simulink subsystem "VehicleElectroThermal"  (R2024b)
settings: Solver=VariableStepAuto  StartTime=0.0  StopTime=10.0  RelTol=1e-3
undefined symbols (not defined in the file): coolant_pipe_D, coolant_valve_D_ratio_max, coolant_valve_D_ratio_min, coolant_valve_displacement, vehicleThermal
libraries: fl_lib x14, SimscapeFluids_lib x6, nesl_utility x6
(part 1 of 2)
Description:
  | This model represents an advanced Battery Electric Vehicle (BEV) architecture with integrated thermal management. It extends the basic electric drivetrain by modeling heat generation, transfer, and cooling subsystems for realistic thermal analysis.
  | 
  | Key Subsystems:
  | • Battery and dual electric motors (Front EM1 and Rear EM2)
  | • Driveline connecting front and rear axles for AWD operation
  | • Thermal components:
  |    - Heater and Chiller for thermal conditioning
  |    - Radiator for external heat rejection
  |    - Battery and Motor Pumps with coolant paths
  |    - Thermal valves and flow routing
  | • HVAC system and DCDC converter for cabin and auxiliary systems
  | • Charger interface for external power input
  | 
  | This Electro-Thermal model enables simulation of temperature effects on vehicle performance and energy consumption, making it ideal for thermal control development, range estimation under thermal load, and energy efficiency studies.
settings Model: Creator=jjha  LastModifiedBy=jjha
settings OptimizationCC: ReuseModelBlockBuffer=off
settings RTWCC: GPUComputeCapability=3.5

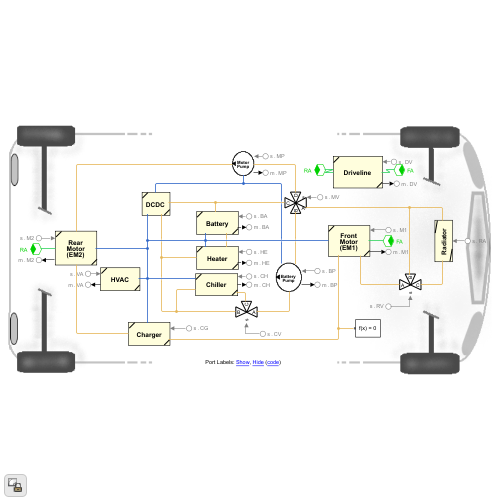
[thumbnail: Simulink's stored preview of the top-level diagram]
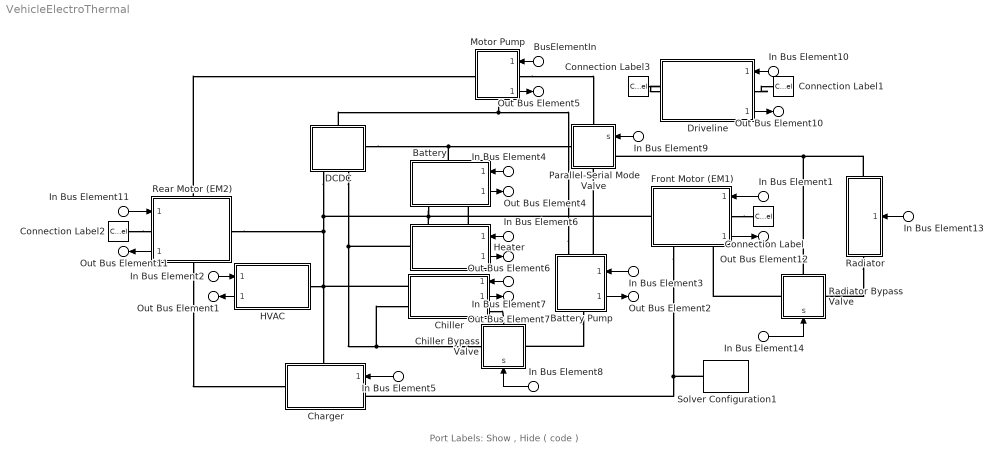
== system VehicleElectroThermal ==
  note: Port Labels: Show , Hide ( code )
  In Bus Element2 : Inport  PortName=s  Element=VA
  In Bus Element3 : Inport  PortName=s  Element=BP
  In Bus Element4 : Inport  PortName=s  Element=BA
  In Bus Element6 : Inport  PortName=s  Element=HE
  In Bus Element7 : Inport  PortName=s  Element=CH
  In Bus Element8 : Inport  PortName=s  Element=CV
  In Bus Element9 : Inport  PortName=s  Element=MV
  In Bus Element10 : Inport  PortName=s  Element=DV
  In Bus Element11 : Inport  PortName=s  Element=M2
  In Bus Element13 : Inport  PortName=s  Element=RA
  In Bus Element14 : Inport  PortName=s  Element=RV
  BusElementIn : Inport  PortName=s  Element=MP
  In Bus Element5 : Inport  PortName=s  Element=CG
  In Bus Element1 : Inport  PortName=s  Element=M1
  Battery : Subsystem  ReferencedSubsystem=BatteryTableBased
      settings: PortSchema="{\"entries\":[{\"content\":{\"sides\":[{\"content\":{\"connectorIds\":[\"In1\",\"Out1\"]},\"type\":\"ConnectorPlacement.EquallySpacedRectSide\",\"uuid\":\"8937d0fc-2bf4-4b6f-a857-82b384a76c94\"},{\"content\":{\"side\":\"RIGHT\"},\"type\":\"ConnectorPlacement.EquallySpacedRectSide\",\"uuid\":\"1ccbeec6-a013-4076-9f98-cb308866a19c\"},{\"content\":{\"connectorIds\":[\"LConn1\"],\"side\":\"TOP\"},\"type\":\"ConnectorPlacement.EquallySpacedRectSide\",\"uuid\":\"77a454e3-c37c-480e-9dd0-9550186f5eb3\"},{\"content\":{\"connectorIds\":[\"RConn1\",\"RConn2\"],\"side\":\"BOTTOM\"},\"type\":\"ConnectorPlacement.EquallySpacedRectSide\",\"uuid\":\"f9a87c6a-7374-41c2-a5df-89d60c915a70\"}]},\"type\":\"ConnectorPlacement.EquallySpacedConnector\",\"uuid\":\"fe008494-fd6d-45a8-bf6b-36872afbad95\"}],\"packageUris\":[\"http://schema.mathworks.com/mf0/Connector/R2020b\"],\"version\":\"1.0\"}"
  Battery Pump : Subsystem  ReferencedSubsystem=Pump  pump_displacement=pump.pump_displacement  pump_speed_max=pump.pump_speed_max  coolant_pipe_D=pump.coolant_pipe_D
      settings: PortSchema="{\"entries\":[{\"content\":{\"sides\":[{\"content\":{\"connectorIds\":[\"In1\",\"Out1\"]},\"type\":\"ConnectorPlacement.EquallySpacedRectSide\",\"uuid\":\"f321ff85-78a4-45a4-ab97-f20c5abfaf5e\"},{\"content\":{\"side\":\"RIGHT\"},\"type\":\"ConnectorPlacement.EquallySpacedRectSide\",\"uuid\":\"2baf3540-3ef2-4140-8c68-0a1895e3ee25\"},{\"content\":{\"connectorIds\":[\"LConn1\",\"LConn2\"],\"side\":\"TOP\"},\"type\":\"ConnectorPlacement.EquallySpacedRectSide\",\"uuid\":\"1e5b09ba-71c5-41d6-b265-2fb2d783e941\"},{\"content\":{\"connectorIds\":[\"RConn1\"],\"side\":\"BOTTOM\"},\"type\":\"ConnectorPlacement.EquallySpacedRectSide\",\"uuid\":\"e2f6a4b1-a05e-4597-9342-cdf640c5f71b\"}]},\"type\":\"ConnectorPlacement.EquallySpacedConnector\",\"uuid\":\"4c01441a-ee4a-4858-900a-4caacc6910c3\"}],\"packageUris\":[\"http://schema.mathworks.com/mf0/Connector/R2020b\"],\"version\":\"1.0\"}"
  Charger : Subsystem  ReferencedSubsystem=ChargerThermalDummy
      settings: PortSchema="{\"entries\":[{\"content\":{\"sides\":[{\"content\":{\"connectorIds\":[\"In1\",\"LConn1\"]},\"type\":\"ConnectorPlacement.EquallySpacedRectSide\",\"uuid\":\"cb45011f-5d5d-4b7e-92e7-7d115d1e4fd6\"},{\"content\":{\"connectorIds\":[\"RConn1\"],\"side\":\"RIGHT\"},\"type\":\"ConnectorPlacement.EquallySpacedRectSide\",\"uuid\":\"cd67087d-6bbf-411e-9f50-cc3c1f5fce85\"},{\"content\":{\"connectorIds\":[\"LConn2\"],\"side\":\"TOP\"},\"type\":\"ConnectorPlacement.EquallySpacedRectSide\",\"uuid\":\"32ff64c9-862a-431f-9f24-2baf455cdab5\"}]},\"type\":\"ConnectorPlacement.EquallySpacedConnector\",\"uuid\":\"13ffd7d0-36a1-4766-a9dc-2d010b2a8713\"}],\"packageUris\":[\"http://schema.mathworks.com/mf0/Connector/R2020b\"],\"version\":\"1.0\"}"
  Chiller : Subsystem  ReferencedSubsystem=Chiller
      settings: PortSchema="{\"entries\":[{\"content\":{\"sides\":[{\"content\":{\"connectorIds\":[\"LConn1\",\"LConn2\"]},\"type\":\"ConnectorPlacement.EquallySpacedRectSide\",\"uuid\":\"5c01cf01-1aa7-4ead-a658-6b31c847d37c\"},{\"content\":{\"connectorIds\":[\"In1\",\"Out1\",\"RConn1\"],\"side\":\"RIGHT\"},\"type\":\"ConnectorPlacement.EquallySpacedRectSide\",\"uuid\":\"fa598d46-0793-4efa-a9e2-c958f5dfdee6\"},{\"content\":{\"side\":\"TOP\"},\"type\":\"ConnectorPlacement.EquallySpacedRectSide\",\"uuid\":\"e82d971a-2580-41ee-87fa-0ab5603b5665\"},{\"content\":{\"side\":\"BOTTOM\"},\"type\":\"ConnectorPlacement.EquallySpacedRectSide\",\"uuid\":\"431a910f-738f-40ab-a4d4-f974d0793b92\"}]},\"type\":\"ConnectorPlacement.EquallySpacedConnector\",\"uuid\":\"9f63eeb1-1768-47e0-a5e5-2e43c100d3fd\"}],\"packageUris\":[\"http://schema.mathworks.com/mf0/Connector/R2020b\"],\"version\":\"1.0\"}"
  Chiller Bypass Valve : Subsystem  Tag=PublishSubsystem
      settings: PortSchema="{\"entries\":[{\"content\":{\"sides\":[{\"content\":{\"connectorIds\":[\"LConn1\"]},\"type\":\"ConnectorPlacement.EquallySpacedRectSide\",\"uuid\":\"3cf8f321-e6af-4e16-922c-cceb23b0b295\"},{\"content\":{\"connectorIds\":[\"In1\"],\"side\":\"RIGHT\"},\"type\":\"ConnectorPlacement.EquallySpacedRectSide\",\"uuid\":\"d134eacd-e7eb-4b63-940a-90eaf4978625\"},{\"content\":{\"connectorIds\":[\"LConn2\"],\"side\":\"TOP\"},\"type\":\"ConnectorPlacement.EquallySpacedRectSide\",\"uuid\":\"57a3d5f7-3b46-4166-b258-196ae00f6810\"},{\"content\":{\"connectorIds\":[\"RConn1\"],\"side\":\"BOTTOM\"},\"type\":\"ConnectorPlacement.EquallySpacedRectSide\",\"uuid\":\"637149da-33c2-49a6-af44-c757a7002402\"}]},\"type\":\"ConnectorPlacement.EquallySpacedConnector\",\"uuid\":\"8ee22012-655b-4352-9f09-996f74687633\"}],\"packageUris\":[\"http://schema.mathworks.com/mf0/Connector/R2020b\"],\"version\":\"1.0\"}"
      mask Display:
      | color('white')
      | plot(100, 100)
      | plot(-100, -100)
      | color('black')
      | 
      | plot([0 -100 -100 0], [0 50 -50 0])
      | plot([0 50 -50 0], [0 100 100 0])
      | plot([0 50 -50 0], [0 -100 -100 0])
  Connection Label : ConnectionLabel  Label=FA
  Connection Label1 : ConnectionLabel  Label=FA
  Connection Label2 : ConnectionLabel  Label=RA
  Connection Label3 : ConnectionLabel  Label=RA
  DCDC : Subsystem  ReferencedSubsystem=PumpDriverTh
      settings: PortSchema="{\"entries\":[{\"content\":{\"sides\":[{\"content\":{\"connectorIds\":[\"RConn2\"]},\"type\":\"ConnectorPlacement.EquallySpacedRectSide\",\"uuid\":\"8937d0fc-2bf4-4b6f-a857-82b384a76c94\"},{\"content\":{\"side\":\"RIGHT\"},\"type\":\"ConnectorPlacement.EquallySpacedRectSide\",\"uuid\":\"1ccbeec6-a013-4076-9f98-cb308866a19c\"},{\"content\":{\"connectorIds\":[\"RConn1\"],\"side\":\"TOP\"},\"type\":\"ConnectorPlacement.EquallySpacedRectSide\",\"uuid\":\"77a454e3-c37c-480e-9dd0-9550186f5eb3\"},{\"content\":{\"connectorIds\":[\"LConn2\",\"LConn1\"],\"side\":\"BOTTOM\"},\"type\":\"ConnectorPlacement.EquallySpacedRectSide\",\"uuid\":\"f9a87c6a-7374-41c2-a5df-89d60c915a70\"}]},\"type\":\"ConnectorPlacement.EquallySpacedConnector\",\"uuid\":\"fe008494-fd6d-45a8-bf6b-36872afbad95\"}],\"packageUris\":[\"http://schema.mathworks.com/mf0/Connector/R2020b\"],\"version\":\"1.0\"}"
  Driveline : Subsystem  ReferencedSubsystem=Driveline
      settings: PortSchema="{\"entries\":[{\"content\":{\"sides\":[{\"content\":{\"connectorIds\":[\"In1\",\"LConn1\",\"Out1\"]},\"type\":\"ConnectorPlacement.EquallySpacedRectSide\",\"uuid\":\"f321ff85-78a4-45a4-ab97-f20c5abfaf5e\"},{\"content\":{\"connectorIds\":[\"RConn1\"],\"side\":\"RIGHT\"},\"type\":\"ConnectorPlacement.EquallySpacedRectSide\",\"uuid\":\"2baf3540-3ef2-4140-8c68-0a1895e3ee25\"},{\"content\":{\"side\":\"TOP\"},\"type\":\"ConnectorPlacement.EquallySpacedRectSide\",\"uuid\":\"1e5b09ba-71c5-41d6-b265-2fb2d783e941\"}]},\"type\":\"ConnectorPlacement.EquallySpacedConnector\",\"uuid\":\"4c01441a-ee4a-4858-900a-4caacc6910c3\"}],\"packageUris\":[\"http://schema.mathworks.com/mf0/Connector/R2020b\"],\"version\":\"1.0\"}"
  Front Motor (EM1) : Subsystem  ReferencedSubsystem=MotorDriveGearTh  max_torque=electricDrive.max_torque  max_power=electricDrive.max_power  Tctc=electricDrive.Tctc  motor_loss_map=electricDrive.motor_loss_map  coolant_channel_D=electricDrive.coolant_channel_D
      settings: PortSchema="{\"entries\":[{\"content\":{\"sides\":[{\"content\":{\"connectorIds\":[\"In1\",\"RConn1\",\"Out1\"]},\"type\":\"ConnectorPlacement.EquallySpacedRectSide\",\"uuid\":\"af07bd2d-3590-42bb-89c7-c9779cf31117\"},{\"content\":{\"connectorIds\":[\"LConn1\"],\"side\":\"RIGHT\"},\"type\":\"ConnectorPlacement.EquallySpacedRectSide\",\"uuid\":\"06bccd0a-b2e1-4e74-ae56-c1e69a7ba035\"},{\"content\":{\"side\":\"TOP\"},\"type\":\"ConnectorPlacement.EquallySpacedRectSide\",\"uuid\":\"3cab1049-b411-40ea-b5ea-dc5d5d9a0e66\"},{\"content\":{\"connectorIds\":[\"LConn2\",\"RConn2\"],\"side\":\"BOTTOM\"},\"type\":\"ConnectorPlacement.EquallySpacedRectSide\",\"uuid\":\"a1b63549-7d05-436f-845e-36a4f25eae53\"}]},\"type\":\"ConnectorPlacement.EquallySpacedConnector\",\"uuid\":\"d2f6dabd-9c76-4b80-9c91-dda4599c36e7\"}],\"packageUris\":[\"http://schema.mathworks.com/mf0/Connector/R2020b\"],\"version\":\"1.0\"}"
  HVAC : Subsystem  ReferencedSubsystem=HVACsimpleTh
      settings: PortSchema="{\"entries\":[{\"content\":{\"sides\":[{\"content\":{\"connectorIds\":[\"LConn1\"]},\"type\":\"ConnectorPlacement.EquallySpacedRectSide\",\"uuid\":\"f3199610-b7b9-4772-9d43-f46decbe6ee9\"},{\"content\":{\"connectorIds\":[\"In1\",\"Out1\"],\"side\":\"RIGHT\"},\"type\":\"ConnectorPlacement.EquallySpacedRectSide\",\"uuid\":\"92399d3a-435b-4545-8fb9-2408b0c62154\"},{\"content\":{\"side\":\"TOP\"},\"type\":\"ConnectorPlacement.EquallySpacedRectSide\",\"uuid\":\"9d5257be-bcde-46da-a005-cbe35149e50d\"},{\"content\":{\"side\":\"BOTTOM\"},\"type\":\"ConnectorPlacement.EquallySpacedRectSide\",\"uuid\":\"da7f19de-1e57-4fc2-b5c3-4c1d680ac086\"}]},\"type\":\"ConnectorPlacement.EquallySpacedConnector\",\"uuid\":\"aa27bbb1-a774-4836-83ea-faf9e12779cd\"}],\"packageUris\":[\"http://schema.mathworks.com/mf0/Connector/R2020b\"],\"version\":\"1.0\"}"
  Heater : Subsystem  ReferencedSubsystem=Heater
      settings: PortSchema="{\"entries\":[{\"content\":{\"sides\":[{\"content\":{},\"type\":\"ConnectorPlacement.EquallySpacedRectSide\",\"uuid\":\"f321ff85-78a4-45a4-ab97-f20c5abfaf5e\"},{\"content\":{\"connectorIds\":[\"RConn1\",\"RConn2\"],\"side\":\"RIGHT\"},\"type\":\"ConnectorPlacement.EquallySpacedRectSide\",\"uuid\":\"2baf3540-3ef2-4140-8c68-0a1895e3ee25\"},{\"content\":{\"connectorIds\":[\"Out1\",\"In1\"],\"side\":\"TOP\"},\"type\":\"ConnectorPlacement.EquallySpacedRectSide\",\"uuid\":\"1e5b09ba-71c5-41d6-b265-2fb2d783e941\"},{\"content\":{\"connectorIds\":[\"RConn3\"],\"side\":\"BOTTOM\"},\"type\":\"ConnectorPlacement.EquallySpacedRectSide\",\"uuid\":\"2993c442-350f-4391-ac34-e98798b669d5\"}]},\"type\":\"ConnectorPlacement.EquallySpacedConnector\",\"uuid\":\"4c01441a-ee4a-4858-900a-4caacc6910c3\"}],\"packageUris\":[\"http://schema.mathworks.com/mf0/Connector/R2020b\"],\"version\":\"1.0\"}"
  Motor Pump : Subsystem  ReferencedSubsystem=Pump  pump_displacement=pump.pump_displacement  pump_speed_max=pump.pump_speed_max  coolant_pipe_D=pump.coolant_pipe_D
      settings: PortSchema="{\"entries\":[{\"content\":{\"sides\":[{\"content\":{\"connectorIds\":[\"In1\",\"LConn1\",\"Out1\"]},\"type\":\"ConnectorPlacement.EquallySpacedRectSide\",\"uuid\":\"f321ff85-78a4-45a4-ab97-f20c5abfaf5e\"},{\"content\":{\"connectorIds\":[\"RConn1\"],\"side\":\"RIGHT\"},\"type\":\"ConnectorPlacement.EquallySpacedRectSide\",\"uuid\":\"2baf3540-3ef2-4140-8c68-0a1895e3ee25\"},{\"content\":{\"side\":\"TOP\"},\"type\":\"ConnectorPlacement.EquallySpacedRectSide\",\"uuid\":\"1e5b09ba-71c5-41d6-b265-2fb2d783e941\"},{\"content\":{\"connectorIds\":[\"LConn2\"],\"side\":\"BOTTOM\"},\"type\":\"ConnectorPlacement.EquallySpacedRectSide\",\"uuid\":\"e2f6a4b1-a05e-4597-9342-cdf640c5f71b\"}]},\"type\":\"ConnectorPlacement.EquallySpacedConnector\",\"uuid\":\"4c01441a-ee4a-4858-900a-4caacc6910c3\"}],\"packageUris\":[\"http://schema.mathworks.com/mf0/Connector/R2020b\"],\"version\":\"1.0\"}"
  Parallel-Serial Mode Valve : Subsystem  Tag=PublishSubsystem
      settings: PortSchema="{\"entries\":[{\"content\":{\"sides\":[{\"content\":{\"connectorIds\":[\"LConn1\"]},\"type\":\"ConnectorPlacement.EquallySpacedRectSide\",\"uuid\":\"37aeff26-8a07-411b-9eeb-30a57d0de01e\"},{\"content\":{\"connectorIds\":[\"RConn1\"],\"side\":\"RIGHT\"},\"type\":\"ConnectorPlacement.EquallySpacedRectSide\",\"uuid\":\"5bec464c-49bf-4ce7-bef9-f1dcc380cec5\"},{\"content\":{\"connectorIds\":[\"LConn2\",\"In1\"],\"side\":\"TOP\"},\"type\":\"ConnectorPlacement.EquallySpacedRectSide\",\"uuid\":\"af2a9b5d-b1fd-40d4-a7a1-24f37b8a323f\"},{\"content\":{\"connectorIds\":[\"RConn2\"],\"side\":\"BOTTOM\"},\"type\":\"ConnectorPlacement.EquallySpacedRectSide\",\"uuid\":\"7361a3ef-1473-4ec0-bd8f-80e79015a6c8\"}]},\"type\":\"ConnectorPlacement.EquallySpacedConnector\",\"uuid\":\"019cf393-57f8-4763-b38e-2892ad46a0e9\"}],\"packageUris\":[\"http://schema.mathworks.com/mf0/Connector/R2020b\"],\"version\":\"1.0\"}"
      mask Display:
      | color('white')
      | plot(100, 100)
      | plot(-100, -100)
      | color('black')
      | 
      | plot([0 -100 -100 0], [0 50 -50 0])
      | plot([0 100 100 0], [0 50 -50 0])
      | plot([0 50 -50 0], [0 100 100 0])
      | plot([0 50 -50 0], [0 -100 -100 0])
  Radiator : Subsystem  ReferencedSubsystem=Radiator
      settings: PortSchema="{\"entries\":[{\"content\":{\"sides\":[{\"content\":{\"connectorIds\":[\"RConn1\"]},\"type\":\"ConnectorPlacement.EquallySpacedRectSide\",\"uuid\":\"af07bd2d-3590-42bb-89c7-c9779cf31117\"},{\"content\":{\"connectorIds\":[\"LConn1\"],\"side\":\"RIGHT\"},\"type\":\"ConnectorPlacement.EquallySpacedRectSide\",\"uuid\":\"06bccd0a-b2e1-4e74-ae56-c1e69a7ba035\"},{\"content\":{\"connectorIds\":[\"In1\"],\"side\":\"TOP\"},\"type\":\"ConnectorPlacement.EquallySpacedRectSide\",\"uuid\":\"3cab1049-b411-40ea-b5ea-dc5d5d9a0e66\"},{\"content\":{\"side\":\"BOTTOM\"},\"type\":\"ConnectorPlacement.EquallySpacedRectSide\",\"uuid\":\"a1b63549-7d05-436f-845e-36a4f25eae53\"}]},\"type\":\"ConnectorPlacement.EquallySpacedConnector\",\"uuid\":\"d2f6dabd-9c76-4b80-9c91-dda4599c36e7\"}],\"packageUris\":[\"http://schema.mathworks.com/mf0/Connector/R2020b\"],\"version\":\"1.0\"}"
  Radiator Bypass Valve : Subsystem  Tag=PublishSubsystem
      settings: PortSchema="{\"entries\":[{\"content\":{\"sides\":[{\"content\":{\"connectorIds\":[\"LConn1\"]},\"type\":\"ConnectorPlacement.EquallySpacedRectSide\",\"uuid\":\"3cf8f321-e6af-4e16-922c-cceb23b0b295\"},{\"content\":{\"connectorIds\":[\"In1\"],\"side\":\"RIGHT\"},\"type\":\"ConnectorPlacement.EquallySpacedRectSide\",\"uuid\":\"d134eacd-e7eb-4b63-940a-90eaf4978625\"},{\"content\":{\"connectorIds\":[\"LConn2\"],\"side\":\"TOP\"},\"type\":\"ConnectorPlacement.EquallySpacedRectSide\",\"uuid\":\"57a3d5f7-3b46-4166-b258-196ae00f6810\"},{\"content\":{\"connectorIds\":[\"RConn1\"],\"side\":\"BOTTOM\"},\"type\":\"ConnectorPlacement.EquallySpacedRectSide\",\"uuid\":\"f8aa24a3-5169-478a-b161-4d226dc0f508\"}]},\"type\":\"ConnectorPlacement.EquallySpacedConnector\",\"uuid\":\"8ee22012-655b-4352-9f09-996f74687633\"}],\"packageUris\":[\"http://schema.mathworks.com/mf0/Connector/R2020b\"],\"version\":\"1.0\"}"
      mask Display:
      | color('white')
      | plot(100, 100)
      | plot(-100, -100)
      | color('black')
      | 
      | plot([0 -100 -100 0], [0 50 -50 0])
      | plot([0 50 -50 0], [0 100 100 0])
      | plot([0 50 -50 0], [0 -100 -100 0])
  Rear Motor (EM2) : Subsystem  ReferencedSubsystem=MotorDriveGearTh  max_torque=electricDrive.max_torque  max_power=electricDrive.max_power  Tctc=electricDrive.Tctc  motor_loss_map=electricDrive.motor_loss_map  coolant_channel_D=electricDrive.coolant_channel_D
      settings: PortSchema="{\"entries\":[{\"content\":{\"sides\":[{\"content\":{\"connectorIds\":[\"In1\",\"RConn1\",\"Out1\"]},\"type\":\"ConnectorPlacement.EquallySpacedRectSide\",\"uuid\":\"af07bd2d-3590-42bb-89c7-c9779cf31117\"},{\"content\":{\"connectorIds\":[\"LConn1\"],\"side\":\"RIGHT\"},\"type\":\"ConnectorPlacement.EquallySpacedRectSide\",\"uuid\":\"06bccd0a-b2e1-4e74-ae56-c1e69a7ba035\"},{\"content\":{\"connectorIds\":[\"LConn2\"],\"side\":\"TOP\"},\"type\":\"ConnectorPlacement.EquallySpacedRectSide\",\"uuid\":\"3cab1049-b411-40ea-b5ea-dc5d5d9a0e66\"},{\"content\":{\"connectorIds\":[\"RConn2\"],\"side\":\"BOTTOM\"},\"type\":\"ConnectorPlacement.EquallySpacedRectSide\",\"uuid\":\"a1b63549-7d05-436f-845e-36a4f25eae53\"}]},\"type\":\"ConnectorPlacement.EquallySpacedConnector\",\"uuid\":\"d2f6dabd-9c76-4b80-9c91-dda4599c36e7\"}],\"packageUris\":[\"http://schema.mathworks.com/mf0/Connector/R2020b\"],\"version\":\"1.0\"}"
  Solver Configuration1 : nesl_utility/Solver Configuration  PhysicalDomain=network_engine_domain  SubClassName=solver  LeftPortType=input  RightPortType=generic  Tones=[]  Harmonics=[]  SimulateNoise=off  Profile=off  UseLocalSampling=off  EnableSwitchedLinearOptims=on  FrequencyDomain=off  UseCCode=off  RelTol=0.001  AbsTol=0.001  MinStep=1e-09  ToWorkspace=off  RevertToSquareIcSolve=off  NumHomotopyIterations=100  PhasorMode=off  PhasorModeNumHarmonics=1  ConsistencySolver=NEWTON_XTOL_AFTER_FTOL  IndexReductionMethod=DerivativeReplacement  DoDC=off  ResidualTolerance=1e-09  ConsistencyTolSource=GLOBAL  ConsistencyAbsTol=0.001  ConsistencyRelTol=0.001  ConsistencyTolFactor=0.001  UseLocalSolver=off  LocalSolverChoice=NE_BACKWARD_EULER_ADVANCER  ResolveIndetEquations=on  FunctionEvalNumThread=1  LocalSolverSampleTime=0.001  DoFixedCost=off  MaxNonlinIter=3  MaxModeIter=2  ComputeImpulses=off  ImpulseIterations=2  LinearAlgebra=auto  LinearAlgebraNumThread=0  EquationFormulation=NE_TIME_EF  DelaysMemoryBudget=1024  AutomaticFiltering=on  FilteringTimeConstant=0.001  PartitionStorageMethod=AS_NEEDED  PartitionMemoryBudget=1024  PartitionMethod=ROBUST  MultibodyUseLocalSolver=off  MultibodyLocalSolverChoice=ODE1  MultibodyLocalSolverSampleTime=0.001
  Out Bus Element1 : Outport  PortName=m  Element=VA
  Out Bus Element2 : Outport  PortName=m  Element=BP
  Out Bus Element4 : Outport  PortName=m  Element=BA
  Out Bus Element6 : Outport  PortName=m  Element=HE
  Out Bus Element7 : Outport  PortName=m  Element=CH
  Out Bus Element10 : Outport  PortName=m  Element=DV
  Out Bus Element11 : Outport  PortName=m  Element=M2
  Out Bus Element12 : Outport  PortName=m  Element=M1
  Out Bus Element5 : Outport  PortName=m  Element=MP
  wires:
  In Bus Element2/1 -> HVAC/1
  In Bus Element6/1 -> Heater/1
  In Bus Element4/1 -> Battery/1
  Chiller/1 -> Out Bus Element7/1
  In Bus Element7/1 -> Chiller/1
  Battery Pump/1 -> Out Bus Element2/1
  BusElementIn/1 -> Motor Pump/1
  In Bus Element3/1 -> Battery Pump/1
  Battery/1 -> Out Bus Element4/1
  HVAC/1 -> Out Bus Element1/1
  In Bus Element8/1 -> Chiller Bypass Valve/1(s)
  In Bus Element9/1 -> Parallel-Serial Mode Valve/1(s)
  Driveline/1 -> Out Bus Element10/1
  In Bus Element10/1 -> Driveline/1
  In Bus Element11/1 -> Rear Motor (EM2)/1
  Rear Motor (EM2)/1 -> Out Bus Element11/1
  Front Motor (EM1)/1 -> Out Bus Element12/1
  In Bus Element13/1 -> Radiator/1
  In Bus Element14/1 -> Radiator Bypass Valve/1(s)
  In Bus Element5/1 -> Charger/1
  Heater/1 -> Out Bus Element6/1
  Motor Pump/1 -> Out Bus Element5/1
  In Bus Element1/1 -> Front Motor (EM1)/1
  connections:
  Radiator Bypass Valve/LConn1 -- Parallel-Serial Mode Valve/LConn2 -- Radiator/LConn1
  Front Motor (EM1)/RConn2 -- Charger/LConn1 -- Solver Configuration1/RConn1
  Chiller Bypass Valve/RConn1 -- DCDC/LConn2 -- Heater/RConn3 -- Chiller/LConn2
  DCDC/RConn2 -- Parallel-Serial Mode Valve/RConn2 -- Battery/LConn1
  Front Motor (EM1)/LConn1 -- Chiller/LConn1 -- Charger/LConn2 -- HVAC/LConn1 -- Rear Motor (EM2)/LConn1 -- DCDC/LConn1 -- Heater/RConn2 -- Battery/RConn2
  Battery Pump/LConn2 -- DCDC/RConn1 -- Motor Pump/LConn2
  Battery Pump/RConn1 -- Chiller Bypass Valve/LConn2
  Motor Pump/LConn1 -- Parallel-Serial Mode Valve/RConn1
  Rear Motor (EM2)/LConn2 -- Motor Pump/RConn1
  Battery Pump/LConn1 -- Parallel-Serial Mode Valve/LConn1
  Rear Motor (EM2)/RConn2 -- Charger/RConn1
  Front Motor (EM1)/RConn1 -- Connection Label/LConn1
  Chiller/RConn1 -- Chiller Bypass Valve/LConn1
  Radiator/RConn1 -- Radiator Bypass Valve/RConn1
  Driveline/LConn1 -- Connection Label1/LConn1
  Connection Label3/LConn1 -- Driveline/RConn1
  Heater/RConn1 -- Battery/RConn1
  Radiator Bypass Valve/LConn2 -- Front Motor (EM1)/LConn2
  Connection Label2/LConn1 -- Rear Motor (EM2)/RConn1

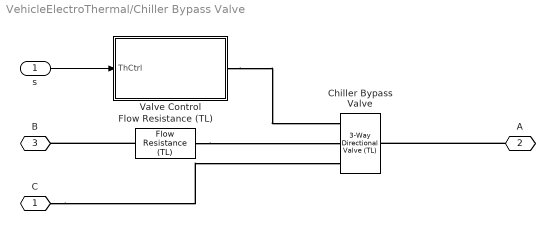
== system VehicleElectroThermal/Chiller Bypass Valve ==
  s : Inport
  Chiller Bypass Valve : SimscapeFluids_lib/Thermal Liquid/Valves & Orifices/Directional Control Valves/3-Way Directional Valve (TL)  open_orifices_pos=fluids.thermal_liquid.valves.directional_control_valves.enum.OpenOrifices3Way.PA  open_orifices_neg=fluids.thermal_liquid.valves.directional_control_valves.enum.OpenOrifices3Way.AT  area_spec=fluids.thermal_liquid.valves.directional_control_valves.enum.area_spec.identical  valve_spec=fluids.thermal_liquid.valves.enum.orifice_spec.linear  del_S_max=vehicleThermal.coolant_valve_displacement-(vehicleThermal.coolant_valve_displacement)*(pi * (vehicleThermal.coolant_valve_D_ratio_min*vehicleThermal.coolant_pipe_D)^2 / 4)/(pi * (vehicleThermal.coolant_valve_D_ratio_max*vehicleThermal.coolant_pipe_D)^2 / 4) m  area_max=pi * (vehicleThermal.coolant_valve_D_ratio_max*vehicleThermal.coolant_pipe_D)^2 / 4 m^2  del_S_TLU=[0 0.002 0.004 0.007 0.017] m  valve_area_TLU=[1e-09, 2.0352e-07, 4.0736e-05, .00011438, .00034356] m^2  del_S_flow_TLU=[0 0.002 0.004 0.007 0.017] m  p_diff_TLU=[-.1, .3, .5, .7] MPa  vol_flow_TLU=1e-3 * [1.7e-05, 2e-05, 2.6e-05; .0035, .0045, .0053; .7, .9, 1.06; 1.96, 2.5, 3; 6, 7.7, 9.13] m^3/s  mdot_TLU=[-1e-05, 1.7e-05, 2e-05, 2.6e-05; -.002, .0035, .0045, .0053; -.4, .7, .9, 1.06; -1.13, 1.96, 2.5, 3; -3.45, 6, 7.7, 9.13] kg/s  T_ref_in=293.15 K  p_ref_in=0.101325 MPa  area_leak=pi * (vehicleThermal.coolant_valve_D_ratio_min*vehicleThermal.coolant_pipe_D)^2 / 4 m^2  Cd=0.7  Re_c=12  smoothing_factor=0.01  pressure_recovery=simscape.enum.onoff.on  area=pi * vehicleThermal.coolant_pipe_D^2 / 4 m^2  S_max_PA=(vehicleThermal.coolant_valve_displacement)*(pi * (vehicleThermal.coolant_valve_D_ratio_min*vehicleThermal.coolant_pipe_D)^2 / 4)/(pi * (vehicleThermal.coolant_valve_D_ratio_max*vehicleThermal.coolant_pipe_D)^2 / 4) - (vehicleThermal.coolant_valve_offset) + vehicleThermal.coolant_valve_displacement-(vehicleThermal.coolant_valve_displacement)*(pi * (vehicleThermal.coolant_valve_D_ratio_min*vehicleThermal.coolant_pipe_D)^2 / 4)/(pi * (vehicleThermal.coolant_valve_D_ratio_max*vehicleThermal.coolant_pipe_D)^2 / 4) m  del_S_max_PA=coolant_valve_displacement-(coolant_valve_displacement)*(pi * (coolant_valve_D_ratio_min*coolant_pipe_D)^2 / 4)/(pi * (coolant_valve_D_ratio_max*coolant_pipe_D)^2 / 4) m  area_max_PA=pi * (coolant_valve_D_ratio_max*coolant_pipe_D)^2 / 4 m^2  del_S_TLU_PA=[0 0.002 0.004 0.007 0.017] m  valve_area_TLU_PA=[1e-09, 2.0352e-07, 4.0736e-05, .00011438, .00034356] m^2  del_S_flow_TLU_PA=[0 0.002 0.004 0.007 0.017] m  p_diff_TLU_PA=[-.1, .3, .5, .7] MPa  vol_flow_TLU_PA=1e-3 * [1.7e-05, 2e-05, 2.6e-05; .0035, .0045, .0053; .7, .9, 1.06; 1.96, 2.5, 3; 6, 7.7, 9.13] m^3/s  mdot_TLU_PA=[-1e-05, 1.7e-05, 2e-05, 2.6e-05; -.002, .0035, .0045, .0053; -.4, .7, .9, 1.06; -1.13, 1.96, 2.5, 3; -3.45, 6, 7.7, 9.13] kg/s  S_max_AT=-(vehicleThermal.coolant_valve_displacement)*(pi * (vehicleThermal.coolant_valve_D_ratio_min*vehicleThermal.coolant_pipe_D)^2 / 4)/(pi * (vehicleThermal.coolant_valve_D_ratio_max*vehicleThermal.coolant_pipe_D)^2 / 4) + (vehicleThermal.coolant_valve_offset) - (vehicleThermal.coolant_valve_displacement-(vehicleThermal.coolant_valve_displacement)*(pi * (vehicleThermal.coolant_valve_D_ratio_min*vehicleThermal.coolant_pipe_D)^2 / 4)/(pi * (vehicleThermal.coolant_valve_D_ratio_max*vehicleThermal.coolant_pipe_D)^2 / 4)) m  del_S_max_AT=coolant_valve_displacement-(coolant_valve_displacement)*(pi * (coolant_valve_D_ratio_min*coolant_pipe_D)^2 / 4)/(pi * (coolant_valve_D_ratio_max*coolant_pipe_D)^2 / 4) m  area_max_AT=pi * (coolant_valve_D_ratio_max*coolant_pipe_D)^2 / 4 m^2  del_S_TLU_AT=[0 0.002 0.004 0.007 0.017] m  valve_area_TLU_AT=[1e-09, 2.0352e-07, 4.0736e-05, .00011438, .00034356] m^2  del_S_flow_TLU_AT=[0 0.002 0.004 0.007 0.017] m  p_diff_TLU_AT=[-.1, .3, .5, .7] MPa  vol_flow_TLU_AT=1e-3 * [1.7e-05, 2e-05, 2.6e-05; .0035, .0045, .0053; .7, .9, 1.06; 1.96, 2.5, 3; 6, 7.7, 9.13] m^3/s  mdot_TLU_AT=[-1e-05, 1.7e-05, 2e-05, 2.6e-05; -.002, .0035, .0045, .0053; -.4, .7, .9, 1.06; -1.13, 1.96, 2.5, 3; -3.45, 6, 7.7, 9.13] kg/s  S_max_PT=2.5e-3 m  del_S_max_PT=0.005 m  area_max_PT=1e-4 m^2  del_S_TLU_PT=[0, .002, .004, .007, .017] m  valve_area_TLU_PT=[1e-09, 2.0352e-07, 4.0736e-05, .00011438, .00034356] m^2  del_S_flow_TLU_PT=[0, .002, .004, .007, .017] m  p_diff_TLU_PT=[.3, .5, .7] MPa  vol_flow_TLU_PT=1e-3 * [1.7e-05, 2e-05, 2.6e-05; .0035, .0045, .0053; .7, .9, 1.06; 1.96, 2.5, 3; 6, 7.7, 9.13] m^3/s  mdot_TLU_PT=[1.7e-05, 2e-05, 2.6e-05; .0035, .0045, .0053; .7, .9, 1.06; 1.96, 2.5, 3; 6, 7.7, 9.13] kg/s
      settings: InternalSimscapePortConfiguration="{\"Bottom\":[],\"Left\":[{\"id\":\"A\",\"label\":\"A\",\"type\":\"foundation.thermal_liquid.thermal_liquid\"}],\"Right\":[{\"id\":\"S\",\"label\":\"S\",\"type\":\"input\"},{\"id\":\"P\",\"label\":\"P\",\"type\":\"foundation.thermal_liquid.thermal_liquid\"},{\"id\":\"T\",\"label\":\"T\",\"type\":\"foundation.thermal_liquid.thermal_liquid\"}],\"Top\":[]}"
  Flow Resistance (TL) : fl_lib/Thermal Liquid/Elements/Flow Resistance (TL)  delta_p_nominal=0.001 MPa  mdot_nominal=0.3 kg/s  area=pi * vehicleThermal.coolant_pipe_D^2 / 4 m^2  laminar_fraction=1e-3
  Valve Control : Subsystem
  C : PMIOPort  Side=Left
  A : PMIOPort  Port=2  Side=Left
  B : PMIOPort  Port=3  Side=Right
  wires:
  s/1 -> Valve Control/1(ThCtrl)
  connections:
  Flow Resistance (TL)/LConn1 -- Chiller Bypass Valve/RConn2
  A/RConn1 -- Chiller Bypass Valve/LConn1
  Valve Control/RConn1 -- Chiller Bypass Valve/RConn1
  C/RConn1 -- Chiller Bypass Valve/RConn3
  Flow Resistance (TL)/RConn1 -- B/RConn1

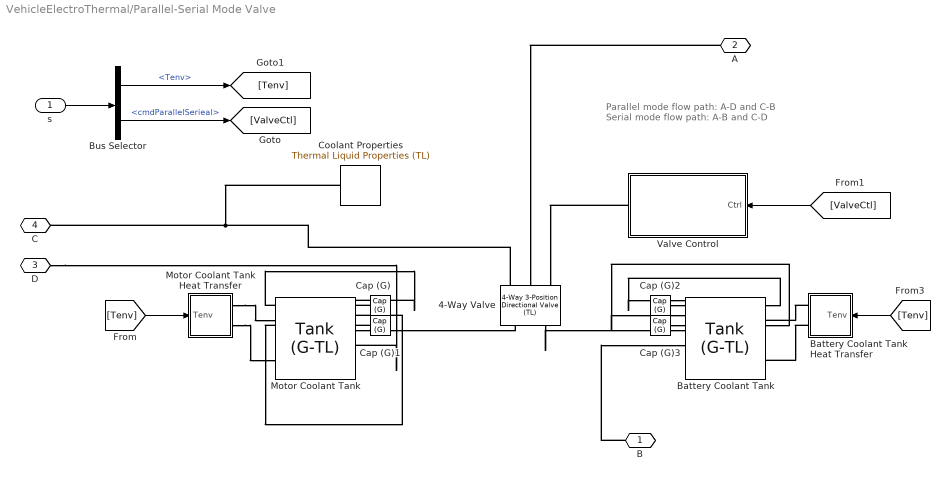
== system VehicleElectroThermal/Parallel-Serial Mode Valve ==
  note: Parallel mode flow path: A-D and C-B
      |
      | Serial mode flow path: A-B and C-D
  s : Inport
  4-Way Valve : SimscapeFluids_lib/Thermal Liquid/Valves & Orifices/Directional Control Valves/4-Way 3-Position Directional Valve (TL)  open_orifices_pos=fluids.thermal_liquid.valves.directional_control_valves.enum.OpenOrifices4WayPosNeg.PA_BT  open_orifices_neu=fluids.thermal_liquid.valves.directional_control_valves.enum.OpenOrifices4WayNeu.all_closed  open_orifices_neg=fluids.thermal_liquid.valves.directional_control_valves.enum.OpenOrifices4WayPosNeg.PB_AT  neutral_assert_action=simscape.enum.assert.action.none  area_spec=fluids.thermal_liquid.valves.directional_control_valves.enum.area_spec.identical  valve_spec=fluids.thermal_liquid.valves.enum.orifice_spec.linear  del_S_max=vehicleThermal.coolant_valve_displacement-(vehicleThermal.coolant_valve_displacement)*(pi * (vehicleThermal.coolant_valve_D_ratio_min*vehicleThermal.coolant_pipe_D)^2 / 4)/(pi * (vehicleThermal.coolant_valve_D_ratio_max*vehicleThermal.coolant_pipe_D)^2 / 4) m  area_max=pi * (vehicleThermal.coolant_valve_D_ratio_max*vehicleThermal.coolant_pipe_D)^2 / 4 m^2  del_S_TLU=[0 0.002 0.004 0.007 0.017] m  valve_area_TLU=[1e-09, 2.0352e-07, 4.0736e-05, .00011438, .00034356] m^2  del_S_flow_TLU=[0 0.002 0.004 0.007 0.017] m  p_diff_TLU=[-.1, .3, .5, .7] MPa  vol_flow_TLU=[-1e-08, 2.2e-08, 2.8e-08, 3.4e-08; -9e-06, .00015, .0002, .00024; -.00036, .00063, .00081, .00096; -.00054, .00094, .0012, .0014; -.00091, .0016, .002, .0024] m^3/s  mdot_TLU=[-1e-05, 1.7e-05, 2e-05, 2.6e-05; -.002, .0035, .0045, .0053; -.4, .7, .9, 1.06; -1.13, 1.96, 2.5, 3; -3.45, 6, 7.7, 9.13] kg/s  p_diff_TLU_const=[-.1, .3, .5, .7] MPa  vol_flow_TLU_const=[-.0009, .0016, .002, .0024] m^3/s  mdot_TLU_const=[-.9, 1.6, 2, 2.4] kg/s  area_const=1e-4 m^2  T_ref_in=293.15 K  p_ref_in=0.101325 MPa  area_leak=pi * (vehicleThermal.coolant_valve_D_ratio_min*vehicleThermal.coolant_pipe_D)^2 / 4 m^2  area=pi * vehicleThermal.coolant_pipe_D^2 / 4 m^2  Cd=0.7  Re_c=12  smoothing_factor=0.01  pressure_recovery=simscape.enum.onoff.on  S_max_PA=(vehicleThermal.coolant_valve_displacement)*(pi * (vehicleThermal.coolant_valve_D_ratio_min*vehicleThermal.coolant_pipe_D)^2 / 4)/(pi * (vehicleThermal.coolant_valve_D_ratio_max*vehicleThermal.coolant_pipe_D)^2 / 4) - (vehicleThermal.coolant_valve_offset) + vehicleThermal.coolant_valve_displacement-(vehicleThermal.coolant_valve_displacement)*(pi * (vehicleThermal.coolant_valve_D_ratio_min*vehicleThermal.coolant_pipe_D)^2 / 4)/(pi * (vehicleThermal.coolant_valve_D_ratio_max*vehicleThermal.coolant_pipe_D)^2 / 4) m  del_S_max_PA=coolant_valve_displacement-(coolant_valve_displacement)*(pi * (coolant_valve_D_ratio_min*coolant_pipe_D)^2 / 4)/(pi * (coolant_valve_D_ratio_max*coolant_pipe_D)^2 / 4) m  area_max_PA=pi * (coolant_valve_D_ratio_max*coolant_pipe_D)^2 / 4 m^2  del_S_TLU_PA=[0 0.002 0.004 0.007 0.017] m  valve_area_TLU_PA=[1e-09, 2.0352e-07, 4.0736e-05, .00011438, .00034356] m^2  del_S_flow_TLU_PA=[0 0.002 0.004 0.007 0.017] m  p_diff_TLU_PA=[-.1, .3, .5, .7] MPa  vol_flow_TLU_PA=[-1e-08, 2.2e-08, 2.8e-08, 3.4e-08; -9e-06, .00015, .0002, .00024; -.00036, .00063, .00081, .00096; -.00054, .00094, .0012, .0014; -.00091, .0016, .002, .0024] m^3/s  mdot_TLU_PA=[-1e-05, 1.7e-05, 2e-05, 2.6e-05; -.002, .0035, .0045, .0053; -.4, .7, .9, 1.06; -1.13, 1.96, 2.5, 3; -3.45, 6, 7.7, 9.13] kg/s  area_const_PA=1e-4 m^2  p_diff_TLU_const_PA=[-.1, .3, .5, .7] MPa  vol_flow_TLU_const_PA=[-.0009, .0016, .002, .0024] m^3/s  mdot_TLU_const_PA=[-.9, 1.6, 2, 2.4] kg/s  S_max_PB=-(vehicleThermal.coolant_valve_displacement)*(pi * (vehicleThermal.coolant_valve_D_ratio_min*vehicleThermal.coolant_pipe_D)^2 / 4)/(pi * (vehicleThermal.coolant_valve_D_ratio_max*vehicleThermal.coolant_pipe_D)^2 / 4) + (vehicleThermal.coolant_valve_offset) - (vehicleThermal.coolant_valve_displacement-(vehicleThermal.coolant_valve_displacement)*(pi * (vehicleThermal.coolant_valve_D_ratio_min*vehicleThermal.coolant_pipe_D)^2 / 4)/(pi * (vehicleThermal.coolant_valve_D_ratio_max*vehicleThermal.coolant_pipe_D)^2 / 4)) m  del_S_max_PB=coolant_valve_displacement-(coolant_valve_displacement)*(pi * (coolant_valve_D_ratio_min*coolant_pipe_D)^2 / 4)/(pi * (coolant_valve_D_ratio_max*coolant_pipe_D)^2 / 4) m  area_max_PB=pi * (coolant_valve_D_ratio_max*coolant_pipe_D)^2 / 4 m^2  del_S_TLU_PB=[0 0.002 0.004 0.007 0.017] m  valve_area_TLU_PB=[1e-09, 2.0352e-07, 4.0736e-05, .00011438, .00034356] m^2  del_S_flow_TLU_PB=[0 0.002 0.004 0.007 0.017] m  p_diff_TLU_PB=[-.1, .3, .5, .7] MPa  vol_flow_TLU_PB=[-1e-08, 2.2e-08, 2.8e-08, 3.4e-08; -9e-06, .00015, .0002, .00024; -.00036, .00063, .00081, .00096; -.00054, .00094, .0012, .0014; -.00091, .0016, .002, .0024] m^3/s  mdot_TLU_PB=[-1e-05, 1.7e-05, 2e-05, 2.6e-05; -.002, .0035, .0045, .0053; -.4, .7, .9, 1.06; -1.13, 1.96, 2.5, 3; -3.45, 6, 7.7, 9.13] kg/s  area_const_PB=1e-4 m^2  p_diff_TLU_const_PB=[-.1, .3, .5, .7] MPa  vol_flow_TLU_const_PB=[-.0009, .0016, .002, .0024] m^3/s  mdot_TLU_const_PB=[-.9, 1.6, 2, 2.4] kg/s  S_max_AB=7.5e-3 m  del_S_max_AB=0.005 m  area_max_AB=1e-4 m^2  del_S_TLU_AB=[0, .00125, .0025, .00375, .005] m  valve_area_TLU_AB=[1e-10, 1e-05, 4e-05, 6e-05, .0001] m^2  del_S_flow_TLU_AB=[0, .00125, .0025, .00375, .005] m  p_diff_TLU_AB=[-.1, .3, .5, .7] MPa  vol_flow_TLU_AB=[-1e-08, 2.2e-08, 2.8e-08, 3.4e-08; -9e-06, .00015, .0002, .00024; -.00036, .00063, .00081, .00096; -.00054, .00094, .0012, .0014; -.00091, .0016, .002, .0024] m^3/s  mdot_TLU_AB=[-1e-05, 1.7e-05, 2e-05, 2.6e-05; -.009, .0035, .0045, .0053; -.36, .7, .9, 1.06; -.54, 1.96, 2.5, 3; -.91, 6, 7.7, 9.13] kg/s  area_const_AB=1e-4 m^2  p_diff_TLU_const_AB=[-.1, .3, .5, .7] MPa  vol_flow_TLU_const_AB=[-.0009, .0016, .002, .0024] m^3/s  mdot_TLU_const_AB=[-.9, 1.6, 2, 2.4] kg/s  S_max_AT=-(vehicleThermal.coolant_valve_displacement)*(pi * (vehicleThermal.coolant_valve_D_ratio_min*vehicleThermal.coolant_pipe_D)^2 / 4)/(pi * (vehicleThermal.coolant_valve_D_ratio_max*vehicleThermal.coolant_pipe_D)^2 / 4) + (vehicleThermal.coolant_valve_offset) - (vehicleThermal.coolant_valve_displacement-(vehicleThermal.coolant_valve_displacement)*(pi * (vehicleThermal.coolant_valve_D_ratio_min*vehicleThermal.coolant_pipe_D)^2 / 4)/(pi * (vehicleThermal.coolant_valve_D_ratio_max*vehicleThermal.coolant_pipe_D)^2 / 4)) m  del_S_max_AT=coolant_valve_displacement-(coolant_valve_displacement)*(pi * (coolant_valve_D_ratio_min*coolant_pipe_D)^2 / 4)/(pi * (coolant_valve_D_ratio_max*coolant_pipe_D)^2 / 4) m  area_max_AT=pi * (coolant_valve_D_ratio_max*coolant_pipe_D)^2 / 4 m^2  del_S_TLU_AT=[0 0.002 0.004 0.007 0.017] m  valve_area_TLU_AT=[1e-09, 2.0352e-07, 4.0736e-05, .00011438, .00034356] m^2  del_S_flow_TLU_AT=[0 0.002 0.004 0.007 0.017] m  p_diff_TLU_AT=[-.1, .3, .5, .7] MPa  vol_flow_TLU_AT=[-1e-08, 2.2e-08, 2.8e-08, 3.4e-08; -9e-06, .00015, .0002, .00024; -.00036, .00063, .00081, .00096; -.00054, .00094, .0012, .0014; -.00091, .0016, .002, .0024] m^3/s  mdot_TLU_AT=[-1e-05, 1.7e-05, 2e-05, 2.6e-05; -.002, .0035, .0045, .0053; -.4, .7, .9, 1.06; -1.13, 1.96, 2.5, 3; -3.45, 6, 7.7, 9.13] kg/s  area_const_AT=1e-4 m^2  p_diff_TLU_const_AT=[-.1, .3, .5, .7] MPa  vol_flow_TLU_const_AT=[-.0009, .0016, .002, .0024] m^3/s  mdot_TLU_const_AT=[-.9, 1.6, 2, 2.4] kg/s  S_max_BT=(vehicleThermal.coolant_valve_displacement)*(pi * (vehicleThermal.coolant_valve_D_ratio_min*vehicleThermal.coolant_pipe_D)^2 / 4)/(pi * (vehicleThermal.coolant_valve_D_ratio_max*vehicleThermal.coolant_pipe_D)^2 / 4) - (vehicleThermal.coolant_valve_offset) + vehicleThermal.coolant_valve_displacement-(vehicleThermal.coolant_valve_displacement)*(pi * (vehicleThermal.coolant_valve_D_ratio_min*vehicleThermal.coolant_pipe_D)^2 / 4)/(pi * (vehicleThermal.coolant_valve_D_ratio_max*vehicleThermal.coolant_pipe_D)^2 / 4) m  del_S_max_BT=coolant_valve_displacement-(coolant_valve_displacement)*(pi * (coolant_valve_D_ratio_min*coolant_pipe_D)^2 / 4)/(pi * (coolant_valve_D_ratio_max*coolant_pipe_D)^2 / 4) m  area_max_BT=pi * (coolant_valve_D_ratio_max*coolant_pipe_D)^2 / 4 m^2  del_S_TLU_BT=[0 0.002 0.004 0.007 0.017] m  valve_area_TLU_BT=[1e-09, 2.0352e-07, 4.0736e-05, .00011438, .00034356] m^2  del_S_flow_TLU_BT=[0 0.002 0.004 0.007 0.017] m  p_diff_TLU_BT=[-.1, .3, .5, .7] MPa  vol_flow_TLU_BT=[-1e-08, 2.2e-08, 2.8e-08, 3.4e-08; -9e-06, .00015, .0002, .00024; -.00036, .00063, .00081, .00096; -.00054, .00094, .0012, .0014; -.00091, .0016, .002, .0024] m^3/s  mdot_TLU_BT=[-1e-05, 1.7e-05, 2e-05, 2.6e-05; -.002, .0035, .0045, .0053; -.4, .7, .9, 1.06; -1.13, 1.96, 2.5, 3; -3.45, 6, 7.7, 9.13] kg/s  area_const_BT=1e-4 m^2  p_diff_TLU_const_BT=[-.1, .3, .5, .7] MPa  vol_flow_TLU_const_BT=[-.0009, .0016, .002, .0024] m^3/s  mdot_TLU_const_BT=[-.9, 1.6, 2, 2.4] kg/s  S_max_PT=0 m  del_S_max_PT=0.005 m  area_max_PT=1e-4 m^2  del_S_TLU_PT=[0, .00125, .0025, .00375, .005] m  valve_area_TLU_PT=[1e-10, 1e-05, 4e-05, 6e-05, .0001] m^2  del_S_flow_TLU_PT=[0, .00125, .0025, .00375, .005] m  p_diff_TLU_PT=[-.1, .3, .5, .7] MPa  vol_flow_TLU_PT=[-1e-08, 2.2e-08, 2.8e-08, 3.4e-08; -9e-06, .00015, .0002, .00024; -.00036, .00063, .00081, .00096; -.00054, .00094, .0012, .0014; -.00091, .0016, .002, .0024] m^3/s  mdot_TLU_PT=[-1e-05, 1.7e-05, 2e-05, 2.6e-05; -.009, .0035, .0045, .0053; -.36, .7, .9, 1.06; -.54, 1.96, 2.5, 3; -.91, 6, 7.7, 9.13] kg/s
      settings: InternalSimscapePortConfiguration="{\"Bottom\":[],\"Left\":[{\"id\":\"A\",\"label\":\"A\",\"type\":\"foundation.thermal_liquid.thermal_liquid\"},{\"id\":\"B\",\"label\":\"B\",\"type\":\"foundation.thermal_liquid.thermal_liquid\"}],\"Right\":[{\"id\":\"S\",\"label\":\"S\",\"type\":\"input\"},{\"id\":\"P\",\"label\":\"P\",\"type\":\"foundation.thermal_liquid.thermal_liquid\"},{\"id\":\"T\",\"label\":\"T\",\"type\":\"foundation.thermal_liquid.thermal_liquid\"}],\"Top\":[]}"
  Battery Coolant Tank : SimscapeFluids_lib/Thermal Liquid/Tanks & Accumulators/Tank (G-TL)  num_inlet=2  volume_total=vehicleThermal.coolant_tank_volume l  volume_spec=1  tank_area=vehicleThermal.coolant_tank_area m^2  level_TLU=[0, 3, 5] m  volume_TLU=[0, 4, 6] m^3  inlet_areas_A1B1=[.01, .01] m^2  inlet_height_A2=0.1 m  inlet_area_A2=0.01 m^2  inlet_heights_A2B2=[0, 0] m  inlet_areas_A2B2=[1 1] * pi * vehicleThermal.coolant_pipe_D^2 / 4 m^2  inlet_heights_A2B2C2=[.1, .1, .1] m  inlet_areas_A2B2C2=[.01, .01, .01] m^2  inlet_heights_A2B2C2D2=0.1 * ones(1, 4) m  inlet_areas_A2B2C2D2=0.01 * ones(1, 4) m^2  inlet_heights_A2B2C2D2E2=0.1 * ones(1, 5) m  inlet_areas_A2B2C2D2E2=0.01 * ones(1, 5) m^2  inlet_heights_A2B2C2D2E2F2=0.1 * ones(1, 6) m  inlet_areas_A2B2C2D2E2F2=0.01 * ones(1, 6) m^2  capacity_check=0  max_liquid_capacity=vehicleThermal.coolant_tank_volume l  g=0 m/s^2  level_specify=on  level_priority=None  level=5 m  level_nominal_specify=off  level_nominal_value=1  level_nominal_unit=m  volume_liquid_specify=on  volume_liquid_priority=High  volume_liquid=0.25 * vehicleThermal.coolant_tank_volume l  volume_liquid_nominal_specify=off  volume_liquid_nominal_value=1  volume_liquid_nominal_unit=m^3  mass_liquid_specify=off  mass_liquid_priority=None  mass_liquid=5e+3 kg  mass_liquid_nominal_specify=off  mass_liquid_nominal_value=1  mass_liquid_nominal_unit=kg  T_liquid_specify=on  T_liquid_priority=High  T_liquid=vehicleThermal.coolant_T_init K  T_liquid_nominal_specify=off  T_liquid_nominal_value=1  T_liquid_nominal_unit=K  p_gas_specify=on  p_gas_priority=High  p_gas=vehicleThermal.coolant_p_init MPa  p_gas_nominal_specify=off  p_gas_nominal_value=1  p_gas_nominal_unit=MPa  T_gas_specify=on  T_gas_priority=High  T_gas=vehicleThermal.coolant_T_init K  T_gas_nominal_specify=off  T_gas_nominal_value=1  T_gas_nominal_unit=K  rho_gas_specify=off  rho_gas_priority=None  rho_gas=1.2 kg/m^3  rho_gas_nominal_specify=off  rho_gas_nominal_value=1  rho_gas_nominal_unit=kg/m^3
      settings: InternalSimscapePortConfiguration="{\"Bottom\":[],\"Left\":[{\"id\":\"A1\",\"label\":\"A1\",\"type\":\"foundation.gas.gas\"},{\"id\":\"B1\",\"label\":\"B1\",\"type\":\"foundation.gas.gas\"},{\"id\":\"A2\",\"label\":\"A2\",\"type\":\"foundation.thermal_liquid.thermal_liquid\"},{\"id\":\"B2\",\"label\":\"B2\",\"type\":\"foundation.thermal_liquid.thermal_liquid\"}],\"Right\":[{\"id\":\"H1\",\"label\":\"H1\",\"type\":\"foundation.thermal.thermal\"},{\"id\":\"H2\",\"label\":\"H2\",\"type\":\"foundation.thermal.thermal\"}],\"Top\":[{\"id\":\"V_out\",\"label\":\"V\",\"type\":\"output\"},{\"id\":\"L_out\",\"label\":\"L\",\"type\":\"output\"}]}"
  Battery Coolant Tank Heat Transfer : Subsystem
      settings: PortSchema="{\"entries\":[{\"content\":{\"sides\":[{\"content\":{\"connectorIds\":[\"LConn1\",\"LConn2\"]},\"type\":\"ConnectorPlacement.EquallySpacedRectSide\",\"uuid\":\"af2bf9aa-b677-43a6-bf9c-06652e963dea\"},{\"content\":{\"connectorIds\":[\"In1\"],\"side\":\"RIGHT\"},\"type\":\"ConnectorPlacement.EquallySpacedRectSide\",\"uuid\":\"0c704f1a-3c3d-4d07-8f67-904e61e89a98\"},{\"content\":{\"connectorIds\":[],\"side\":\"TOP\"},\"type\":\"ConnectorPlacement.EquallySpacedRectSide\",\"uuid\":\"52658d1d-07bf-431f-9b4a-6993d458b631\"}]},\"type\":\"ConnectorPlacement.EquallySpacedConnector\",\"uuid\":\"47040c62-06d3-42ab-8efb-80a2d029155c\"}],\"packageUris\":[\"http://schema.mathworks.com/mf0/Connector/R2020b\"],\"version\":\"1.0\"}"
  Bus Selector : BusSelector  OutputSignals=Tenv,cmdParallelSerieal
  Cap (G){,1..3} (4 alike) : fl_lib/Gas/Elements/Cap (G)  p_specify=off  p_priority=None  p=0.101325 MPa  p_nominal_specify=off  p_nominal_value=1  p_nominal_unit=MPa  T_specify=off  T_priority=None  T=293.15 K  T_nominal_specify=off  T_nominal_value=1  T_nominal_unit=K
  Coolant Properties : SimscapeFluids_lib/Thermal Liquid/Utilities/Thermal Liquid Properties (TL)  fluid_list=fluids.thermal_liquid.utilities.enum.thermal_liquid_fluid_list.ethylene_glycol  concentration_param_EG=fluids.thermal_liquid.utilities.enum.thermal_liquid_concentration.volume_fraction  concentration_param_PG=fluids.thermal_liquid.utilities.enum.thermal_liquid_concentration.volume_fraction  c_mass_SW=3.5e-3  c_mass_EG=0.1  c_mass_PG=0.1  c_mass_GL=0.1  c_vol_EG=0.5  c_vol_PG=0.1  beta_const_EG=2.1791 GPa  beta_const_PG=2.1791 GPa  beta_const_GL=2.1791 GPa  p_min_EG=0.01 MPa  p_min_PG=0.01 MPa  p_min_GL=0.01 MPa  p_max_EG=50 MPa  p_max_PG=50 MPa  p_max_GL=50 MPa  p_atm=0.101325 MPa  properties_range_check=simscape.enum.assert.action.error
  Motor Coolant Tank : SimscapeFluids_lib/Thermal Liquid/Tanks & Accumulators/Tank (G-TL)  num_inlet=2  volume_total=vehicleThermal.coolant_tank_volume l  volume_spec=1  tank_area=vehicleThermal.coolant_tank_area m^2  level_TLU=[0, 3, 5] m  volume_TLU=[0, 4, 6] m^3  inlet_areas_A1B1=[.01, .01] m^2  inlet_height_A2=0.1 m  inlet_area_A2=0.01 m^2  inlet_heights_A2B2=[0, 0] m  inlet_areas_A2B2=[1 1] * pi * vehicleThermal.coolant_pipe_D^2 / 4 m^2  inlet_heights_A2B2C2=[.1, .1, .1] m  inlet_areas_A2B2C2=[.01, .01, .01] m^2  inlet_heights_A2B2C2D2=0.1 * ones(1, 4) m  inlet_areas_A2B2C2D2=0.01 * ones(1, 4) m^2  inlet_heights_A2B2C2D2E2=0.1 * ones(1, 5) m  inlet_areas_A2B2C2D2E2=0.01 * ones(1, 5) m^2  inlet_heights_A2B2C2D2E2F2=0.1 * ones(1, 6) m  inlet_areas_A2B2C2D2E2F2=0.01 * ones(1, 6) m^2  capacity_check=0  max_liquid_capacity=vehicleThermal.coolant_tank_volume l  g=0 m/s^2  level_specify=on  level_priority=None  level=5 m  level_nominal_specify=off  level_nominal_value=1  level_nominal_unit=m  volume_liquid_specify=on  volume_liquid_priority=High  volume_liquid=0.25 * vehicleThermal.coolant_tank_volume l  volume_liquid_nominal_specify=off  volume_liquid_nominal_value=1  volume_liquid_nominal_unit=m^3  mass_liquid_specify=off  mass_liquid_priority=None  mass_liquid=5e+3 kg  mass_liquid_nominal_specify=off  mass_liquid_nominal_value=1  mass_liquid_nominal_unit=kg  T_liquid_specify=on  T_liquid_priority=High  T_liquid=vehicleThermal.coolant_T_init K  T_liquid_nominal_specify=off  T_liquid_nominal_value=1  T_liquid_nominal_unit=K  p_gas_specify=on  p_gas_priority=High  p_gas=vehicleThermal.coolant_p_init MPa  p_gas_nominal_specify=off  p_gas_nominal_value=1  p_gas_nominal_unit=MPa  T_gas_specify=on  T_gas_priority=High  T_gas=vehicleThermal.coolant_T_init K  T_gas_nominal_specify=off  T_gas_nominal_value=1  T_gas_nominal_unit=K  rho_gas_specify=off  rho_gas_priority=None  rho_gas=1.2 kg/m^3  rho_gas_nominal_specify=off  rho_gas_nominal_value=1  rho_gas_nominal_unit=kg/m^3
      settings: InternalSimscapePortConfiguration="{\"Bottom\":[],\"Left\":[{\"id\":\"A1\",\"label\":\"A1\",\"type\":\"foundation.gas.gas\"},{\"id\":\"B1\",\"label\":\"B1\",\"type\":\"foundation.gas.gas\"},{\"id\":\"A2\",\"label\":\"A2\",\"type\":\"foundation.thermal_liquid.thermal_liquid\"},{\"id\":\"B2\",\"label\":\"B2\",\"type\":\"foundation.thermal_liquid.thermal_liquid\"}],\"Right\":[{\"id\":\"H1\",\"label\":\"H1\",\"type\":\"foundation.thermal.thermal\"},{\"id\":\"H2\",\"label\":\"H2\",\"type\":\"foundation.thermal.thermal\"}],\"Top\":[{\"id\":\"V_out\",\"label\":\"V\",\"type\":\"output\"},{\"id\":\"L_out\",\"label\":\"L\",\"type\":\"output\"}]}"
  Motor Coolant Tank Heat Transfer : Subsystem
  Valve Control : Subsystem
  B : PMIOPort  Side=Left
  A : PMIOPort  Port=2  Side=Left
  D : PMIOPort  Port=3  Side=Right
  C : PMIOPort  Port=4  Side=Right
  wires:
  Bus Selector/2 -> [ValveCtl]  "<cmdParallelSerieal>"
  Bus Selector/1 -> [Tenv]  "<Tenv>"
  s/1 -> Bus Selector/1
  [ValveCtl] -> Valve Control/1(Ctrl)
  [Tenv] -> Battery Coolant Tank Heat Transfer/1(Tenv)
  [Tenv] -> Motor Coolant Tank Heat Transfer/1(Tenv)
  connections:
  Battery Coolant Tank Heat Transfer/LConn2 -- Battery Coolant Tank/RConn2
  Battery Coolant Tank Heat Transfer/LConn1 -- Battery Coolant Tank/RConn1
  D/RConn1 -- Motor Coolant Tank/LConn4
  Cap (G)/LConn1 -- Motor Coolant Tank/LConn1
  Motor Coolant Tank Heat Transfer/RConn2 -- Motor Coolant Tank/RConn2
  Motor Coolant Tank/LConn3 -- 4-Way Valve/LConn2
  Cap (G)2/LConn1 -- Battery Coolant Tank/LConn1
  Cap (G)3/LConn1 -- Battery Coolant Tank/LConn2
  Motor Coolant Tank Heat Transfer/RConn1 -- Motor Coolant Tank/RConn1
  Cap (G)1/LConn1 -- Motor Coolant Tank/LConn2
  4-Way Valve/LConn1 -- Battery Coolant Tank/LConn3
  Valve Control/RConn1 -- 4-Way Valve/RConn1
  B/RConn1 -- Battery Coolant Tank/LConn4
  A/RConn1 -- 4-Way Valve/RConn2
  4-Way Valve/RConn3 -- C/RConn1 -- Coolant Properties/RConn1
